simulink model "untitled"  (R2016a)
settings: Solver=VariableStepAuto  StartTime=0.0  StopTime=10.0  RelTol=1e-3
settings Model: Creator=Shinelon  LastModifiedBy=Shinelon

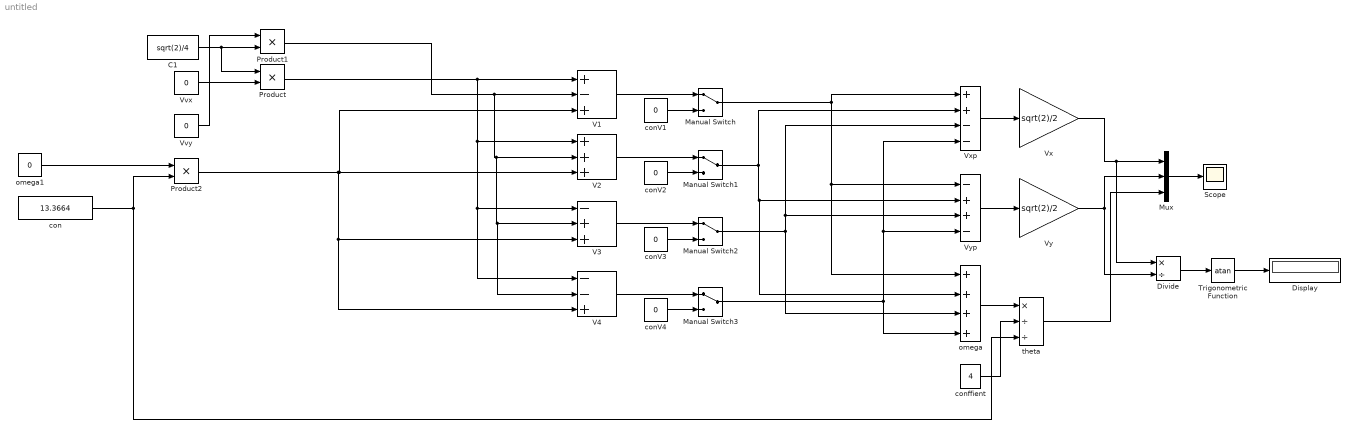
== system untitled ==
  "C1 " : Constant  Value=sqrt(2)/4
  Display : Display
  Divide : Product  Inputs=*/
  Manual Switch{,1..3} (4 alike) : ManualSwitch
  Mux : Mux  Inputs=3
  Product : Product
  Product1 : Product
  Product2 : Product
  Scope : Scope
  Trigonometric Function : Trigonometry  Operator=atan  OutputSignalType=real
  "V1 " : Sum  Inputs=+-+
  V2 : Sum  Inputs=+++
  V3 : Sum  Inputs=-++
  V4 : Sum  Inputs=--+
  "Vvx " : Constant  Value=0
  "Vvy " : Constant  Value=0
  "Vx " : Gain  Gain=sqrt(2)/2
  Vxp : Sum  Inputs=++--
  "Vy " : Gain  Gain=sqrt(2)/2
  "Vyp " : Sum  Inputs=-++-
  "con " : Constant  Value=13.3664
  conV1 : Constant  Value=0
  conV2 : Constant  Value=0
  conV3 : Constant  Value=0
  "conV4 " : Constant  Value=0
  "conffient " : Constant  Value=4
  "omega " : Sum  Inputs=++++
  "omega1 " : Constant  Value=0
  theta : Product  Inputs=*//
  wires:
  V4/1 -> Manual Switch3/1
  Vxp/1 -> "Vx "/1
  "Vyp "/1 -> "Vy "/1
  Mux/1 -> Scope/1
  "Vx "/1 -> Mux/1, Divide/1
  "Vy "/1 -> Divide/2, Mux/2
  Divide/1 -> Trigonometric Function/1
  Trigonometric Function/1 -> Display/1
  "omega "/1 -> theta/1
  "conffient "/1 -> theta/2
  "con "/1 -> theta/3, Product2/2
  theta/1 -> Mux/3
  Manual Switch3/1 -> "omega "/4, "Vyp "/4, Vxp/4
  "conV4 "/1 -> Manual Switch3/2
  conV3/1 -> Manual Switch2/2
  Manual Switch2/1 -> "omega "/3, "Vyp "/3, Vxp/3
  V3/1 -> Manual Switch2/1
  conV2/1 -> Manual Switch1/2
  V2/1 -> Manual Switch1/1
  Manual Switch1/1 -> Vxp/2, "omega "/2, "Vyp "/2
  conV1/1 -> Manual Switch/2
  Manual Switch/1 -> Vxp/1, "Vyp "/1, "omega "/1
  "V1 "/1 -> Manual Switch/1
  "C1 "/1 -> Product1/2, Product/1
  "Vvx "/1 -> Product/2
  Product/1 -> V4/1, V3/1, V2/1, "V1 "/1
  "Vvy "/1 -> Product1/1
  Product1/1 -> V4/2, V3/2, V2/2, "V1 "/2
  "omega1 "/1 -> Product2/1
  Product2/1 -> V4/3, V3/3, "V1 "/3, V2/3
